simulink model "VSC_GFo_Fixed_Frequency_wi_LCL_v2017b"  (R2017b)
settings: Solver=ode1  StartTime=0.0  StopTime=10  FixedStep=Time_Step  MaxStep=1e-5  RelTol=1e-3
values from neighbouring files (symbols this model uses):
  fb = fn    (= 50)    [VSC_GFo_Init.m]    (also in VSC_GFo_Init_v1.m; VSC_GFo_Init_wi_LCL.m)
  fn = 50    [VSC_GFo_Init.m]    (also in VSC_GFo_Init_v1.m; VSC_GFo_Init_wi_LCL.m)
  GRD00_H = 5    [VSC_GFo_Init.m]    (also in VSC_GFo_Init_v1.m; VSC_GFo_Init_wi_LCL.m)
  GRD00_R = 4/100    (= 0.04)    [VSC_GFo_Init.m]    (also in VSC_GFo_Init_v1.m; VSC_GFo_Init_wi_LCL.m)
  GRD00_TD = 6    [VSC_GFo_Init.m]    (also in VSC_GFo_Init_v1.m = 2; VSC_GFo_Init_wi_LCL.m = 2)
  GRD00_TN = 1    [VSC_GFo_Init.m]    (also in VSC_GFo_Init_v1.m; VSC_GFo_Init_wi_LCL.m)
  GRD00_Ub = GRD00_Un    (= 400000)    [VSC_GFo_Init.m]    (also in VSC_GFo_Init_v1.m; VSC_GFo_Init_wi_LCL.m)
  Time_Step = 40e-6    (= 4e-05)    [VSC_GFo_Init.m]    (also in VSC_GFo_Init_v1.m; VSC_GFo_Init_wi_LCL.m)
  VSC01_Cf_pu = 0.066    [VSC_GFo_Init.m]    (also in VSC_GFo_Init_wi_LCL.m)
  VSC01_Lf_pu = 0.15    [VSC_GFo_Init.m]    (also in VSC_GFo_Init_wi_LCL.m)
  VSC01_Lt_pu = 0.15    [VSC_GFo_Init.m]    (also in VSC_GFo_Init_v1.m; VSC_GFo_Init_wi_LCL.m)
  VSC01_mp1 = 0.0043    [VSC_GFo_Init.m]    (also in VSC_GFo_Init_v1.m; VSC_GFo_Init_wi_LCL.m)
  VSC01_mp2 = 0.003    [VSC_GFo_Init.m]    (also in VSC_GFo_Init_v1.m = 0.0033; VSC_GFo_Init_wi_LCL.m = 0.0033)
  VSC01_mp3 = 0.04    [VSC_GFo_Init.m]    (also in VSC_GFo_Init_v1.m; VSC_GFo_Init_wi_LCL.m)
  VSC01_Pn = 1000 * 1e6    (= 1000000000)    [VSC_GFo_Init.m]    (also in VSC_GFo_Init_v1.m; VSC_GFo_Init_wi_LCL.m)
  VSC01_R = 4/100    (= 0.04)    [VSC_GFo_Init.m]    (also in VSC_GFo_Init_v1.m; VSC_GFo_Init_wi_LCL.m)
  VSC01_Rt_pu = 0.005    [VSC_GFo_Init.m]    (also in VSC_GFo_Init_v1.m; VSC_GFo_Init_wi_LCL.m)
  VSC01_Rv = 0.09    [VSC_GFo_Init.m]    (also in VSC_GFo_Init_v1.m; VSC_GFo_Init_wi_LCL.m)
  VSC01_Sn = VSC01_Pn/VSC01_cosPhi_n    [VSC_GFo_Init.m]    (also in VSC_GFo_Init_v1.m; VSC_GFo_Init_wi_LCL.m)
  VSC01_T1 = 0.121    [VSC_GFo_Init.m]    (also in VSC_GFo_Init_v1.m; VSC_GFo_Init_wi_LCL.m)
  VSC01_T2 = 0.022    [VSC_GFo_Init.m]    (also in VSC_GFo_Init_v1.m; VSC_GFo_Init_wi_LCL.m)
  VSC01_Tr_PLL = 0.010    (= 0.01)    [VSC_GFo_Init.m]    (also in VSC_GFo_Init_v1.m; VSC_GFo_Init_wi_LCL.m)
  VSC01_Udc_n = 640 * 1e3    (= 640000)    [VSC_GFo_Init.m]    (also in VSC_GFo_Init_v1.m; VSC_GFo_Init_wi_LCL.m)
  VSC01_Udcb = VSC01_Udc_n    (= 640000)    [VSC_GFo_Init.m]    (also in VSC_GFo_Init_v1.m; VSC_GFo_Init_wi_LCL.m)
  VSC01_Un1 = 320 * 1e3    (= 320000)    [VSC_GFo_Init.m]    (also in VSC_GFo_Init_v1.m; VSC_GFo_Init_wi_LCL.m)
  VSC01_Un2 = 400 * 1e3    (= 400000)    [VSC_GFo_Init.m]    (also in VSC_GFo_Init_v1.m; VSC_GFo_Init_wi_LCL.m)
  VSC01_W_LF = 60    [VSC_GFo_Init.m]    (also in VSC_GFo_Init_v1.m; VSC_GFo_Init_wi_LCL.m)
  VSC01_wc1 = wb/10    (= 31.4159265359)    [VSC_GFo_Init.m]    (also in VSC_GFo_Init_v1.m; VSC_GFo_Init_wi_LCL.m)
  VSC01_wc2 = 33.3    [VSC_GFo_Init.m]    (also in VSC_GFo_Init_v1.m; VSC_GFo_Init_wi_LCL.m)
  VSC01_wc3 = 2.5    [VSC_GFo_Init.m]    (also in VSC_GFo_Init_v1.m; VSC_GFo_Init_wi_LCL.m)
undefined symbols (not defined in the file or in its folder): C_line, VSC01_id0
libraries: powerlib x31, powerlib_meascontrol x1
(part 3 of 3)

== system VSC_GFo_Fixed_Frequency_wi_LCL_v2017b/VSC00/Strategy 1/Inner controller: Current & Voltage /Current Control/PI current control axis d1 ==
  e : Inport
  x0 : Inport  Port=2
  Damping (d) : Gain  Gain=Kp_i
  Damping (d)1 : Gain  Gain=1/Kp_i
  Integration Time : Gain  Gain=1/Ti_i
  Integrator : Integrator  InitialConditionSource=external
  Sum1 : Sum  Inputs=|++
  Sum2 : Sum  Inputs=-+|
  v_q : Outport
  wires:
  Damping (d)/1 -> v_q/1  "v_d\""
  e/1 -> Integration Time/1, Sum1/2, Sum2/1
  Sum1/1 -> Damping (d)/1
  Integrator/1 -> Sum1/1
  Integration Time/1 -> Integrator/1
  x0/1 -> Damping (d)1/1
  Damping (d)1/1 -> Sum2/2
  Sum2/1 -> Integrator/2

== system VSC_GFo_Fixed_Frequency_wi_LCL_v2017b/VSC00/Strategy 1/Inner controller: Current & Voltage /Voltage Control/PI voltage control axis d ==
  e : Inport
  x0 : Inport  Port=2
  Damping (d) : Gain  Gain=Kp_v
  Damping (d)1 : Gain  Gain=1/Kp_v
  Integration Time : Gain  Gain=1/Ti_iv
  Integrator : Integrator  InitialConditionSource=external
  Sum1 : Sum  Inputs=|++
  Sum2 : Sum  Inputs=-+|
  is_d'' : Outport
  wires:
  Integration Time/1 -> Integrator/1
  Integrator/1 -> Sum1/1
  Sum1/1 -> Damping (d)/1
  Damping (d)/1 -> is_d''/1  "Is_d\""
  Damping (d)1/1 -> Sum2/2
  e/1 -> Sum2/1, Sum1/2, Integration Time/1
  Sum2/1 -> Integrator/2
  x0/1 -> Damping (d)1/1

== system VSC_GFo_Fixed_Frequency_wi_LCL_v2017b/VSC00/Strategy 1/Inner controller: Current & Voltage /Voltage Control/PI voltage control axis d1 ==
  e : Inport
  x0 : Inport  Port=2
  Damping (d) : Gain  Gain=Kp_v
  Damping (d)1 : Gain  Gain=1/Kp_v
  Integration Time : Gain  Gain=1/Ti_iv
  Integrator : Integrator  InitialConditionSource=external
  Sum1 : Sum  Inputs=|++
  Sum2 : Sum  Inputs=-+|
  is_d'' : Outport
  wires:
  Integration Time/1 -> Integrator/1
  Integrator/1 -> Sum1/1
  Sum1/1 -> Damping (d)/1
  Damping (d)/1 -> is_d''/1  "Is_d\""
  Damping (d)1/1 -> Sum2/2
  e/1 -> Sum2/1, Sum1/2, Integration Time/1
  Sum2/1 -> Integrator/2
  x0/1 -> Damping (d)1/1

== system VSC_GFo_Fixed_Frequency_wi_LCL_v2017b/VSC00/Strategy 1/Park Transformation_abc--> dq0/abc --> dq1/abc_alpha_beta_tri4 ==
  a : Inport
  b : Inport  Port=2
  c : Inport  Port=3
  Fcn1 : Fcn  Expr=sqrt(2/3)*(u(1)+u(2)+u(3))
  Fcn3 : Fcn  Expr=sqrt(2/3)*(u(1)-u(2)/2-u(3)/2)
  Fcn5 : Fcn  Expr=(u(2)-u(3))/sqrt(2)
  Mux : Mux  Inputs=3
  Scope5 : Scope
  alpha : Outport
  beta : Outport  Port=2
  wires:
  Fcn5/1 -> beta/1
  Fcn3/1 -> alpha/1
  b/1 -> Mux/2
  a/1 -> Mux/1
  Mux/1 -> Fcn3/1, Fcn1/1, Fcn5/1
  Fcn1/1 -> Scope5/1
  c/1 -> Mux/3

== system VSC_GFo_Fixed_Frequency_wi_LCL_v2017b/VSC00/Strategy 1/Park Transformation_abc--> dq0/abc --> dq1/abc_dq2 ==
  Theta : Inport
  a : Inport  Port=2
  b : Inport  Port=3
  1/Vb1 : Gain  Gain=1/(sqrt(3))
  1/Vb2 : Gain  Gain=1/(sqrt(3))
  Fcn1 : Fcn  Expr=u(2)*cos(u(1))+u(3)*sin(u(1))
  Fcn3 : Fcn  Expr=u(2)*sin(u(1))-u(3)*cos(u(1))
  Mux : Mux  Inputs=3
  d : Outport
  q : Outport  Port=2
  wires:
  1/Vb2/1 -> q/1
  1/Vb1/1 -> d/1
  Fcn1/1 -> 1/Vb2/1
  Fcn3/1 -> 1/Vb1/1
  b/1 -> Mux/3
  a/1 -> Mux/2
  Mux/1 -> Fcn1/1, Fcn3/1
  Theta/1 -> Mux/1

== system VSC_GFo_Fixed_Frequency_wi_LCL_v2017b/VSC00/Strategy 1/Park Transformation_abc--> dq0/abc --> dq2/abc_alpha_beta_tri4 ==
  a : Inport
  b : Inport  Port=2
  c : Inport  Port=3
  Fcn1 : Fcn  Expr=sqrt(2/3)*(u(1)+u(2)+u(3))
  Fcn3 : Fcn  Expr=sqrt(2/3)*(u(1)-u(2)/2-u(3)/2)
  Fcn5 : Fcn  Expr=(u(2)-u(3))/sqrt(2)
  Mux : Mux  Inputs=3
  Scope5 : Scope
  alpha : Outport
  beta : Outport  Port=2
  wires:
  c/1 -> Mux/3
  Fcn1/1 -> Scope5/1
  Mux/1 -> Fcn5/1, Fcn1/1, Fcn3/1
  a/1 -> Mux/1
  b/1 -> Mux/2
  Fcn3/1 -> alpha/1
  Fcn5/1 -> beta/1

== system VSC_GFo_Fixed_Frequency_wi_LCL_v2017b/VSC00/Strategy 1/Park Transformation_abc--> dq0/abc --> dq2/abc_dq2 ==
  Theta : Inport
  a : Inport  Port=2
  b : Inport  Port=3
  1/Vb1 : Gain  Gain=1/(sqrt(3))
  1/Vb2 : Gain  Gain=1/(sqrt(3))
  Fcn1 : Fcn  Expr=u(2)*cos(u(1))+u(3)*sin(u(1))
  Fcn3 : Fcn  Expr=u(2)*sin(u(1))-u(3)*cos(u(1))
  Mux : Mux  Inputs=3
  d : Outport
  q : Outport  Port=2
  wires:
  Theta/1 -> Mux/1
  Mux/1 -> Fcn3/1, Fcn1/1
  a/1 -> Mux/2
  b/1 -> Mux/3
  Fcn3/1 -> 1/Vb1/1
  Fcn1/1 -> 1/Vb2/1
  1/Vb1/1 -> d/1
  1/Vb2/1 -> q/1

== system VSC_GFo_Fixed_Frequency_wi_LCL_v2017b/VSC00/Strategy 1/Park Transformation_abc--> dq0/abc --> dq4/abc_alpha_beta_tri4 ==
  a : Inport
  b : Inport  Port=2
  c : Inport  Port=3
  Fcn1 : Fcn  Expr=sqrt(2/3)*(u(1)+u(2)+u(3))
  Fcn3 : Fcn  Expr=sqrt(2/3)*(u(1)-u(2)/2-u(3)/2)
  Fcn5 : Fcn  Expr=(u(2)-u(3))/sqrt(2)
  Mux : Mux  Inputs=3
  Scope5 : Scope
  alpha : Outport
  beta : Outport  Port=2
  wires:
  c/1 -> Mux/3
  Fcn1/1 -> Scope5/1
  Mux/1 -> Fcn5/1, Fcn1/1, Fcn3/1
  a/1 -> Mux/1
  b/1 -> Mux/2
  Fcn3/1 -> alpha/1
  Fcn5/1 -> beta/1

== system VSC_GFo_Fixed_Frequency_wi_LCL_v2017b/VSC00/Strategy 1/Park Transformation_abc--> dq0/abc --> dq4/abc_dq2 ==
  Theta : Inport
  a : Inport  Port=2
  b : Inport  Port=3
  1/Vb1 : Gain  Gain=1/(sqrt(3))
  1/Vb2 : Gain  Gain=1/(sqrt(3))
  Fcn1 : Fcn  Expr=u(2)*cos(u(1))+u(3)*sin(u(1))
  Fcn3 : Fcn  Expr=u(2)*sin(u(1))-u(3)*cos(u(1))
  Mux : Mux  Inputs=3
  d : Outport
  q : Outport  Port=2
  wires:
  Theta/1 -> Mux/1
  Mux/1 -> Fcn3/1, Fcn1/1
  a/1 -> Mux/2
  b/1 -> Mux/3
  Fcn3/1 -> 1/Vb1/1
  Fcn1/1 -> 1/Vb2/1
  1/Vb1/1 -> d/1
  1/Vb2/1 -> q/1

== system VSC_GFo_Fixed_Frequency_wi_LCL_v2017b/VSC00/Strategy 2/Inner controller: Current & Voltage /Current Control/PI current control axis d ==
  e : Inport
  x0 : Inport  Port=2
  Damping (d) : Gain  Gain=Kp_i
  Damping (d)1 : Gain  Gain=1/Kp_i
  Integration Time : Gain  Gain=1/Ti_i
  Integrator : Integrator  InitialConditionSource=external
  Sum1 : Sum  Inputs=|++
  Sum2 : Sum  Inputs=-+|
  v_d'' : Outport
  wires:
  Damping (d)/1 -> v_d''/1  "v_d"
  e/1 -> Integration Time/1, Sum1/2, Sum2/1
  Sum1/1 -> Damping (d)/1
  Integrator/1 -> Sum1/1
  Integration Time/1 -> Integrator/1
  x0/1 -> Damping (d)1/1
  Damping (d)1/1 -> Sum2/2
  Sum2/1 -> Integrator/2

== system VSC_GFo_Fixed_Frequency_wi_LCL_v2017b/VSC00/Strategy 2/Inner controller: Current & Voltage /Current Control/PI current control axis d1 ==
  e : Inport
  x0 : Inport  Port=2
  Damping (d) : Gain  Gain=Kp_i
  Damping (d)1 : Gain  Gain=1/Kp_i
  Integration Time : Gain  Gain=1/Ti_i
  Integrator : Integrator  InitialConditionSource=external
  Sum1 : Sum  Inputs=|++
  Sum2 : Sum  Inputs=-+|
  v_q : Outport
  wires:
  Damping (d)/1 -> v_q/1  "v_d\""
  e/1 -> Integration Time/1, Sum1/2, Sum2/1
  Sum1/1 -> Damping (d)/1
  Integrator/1 -> Sum1/1
  Integration Time/1 -> Integrator/1
  x0/1 -> Damping (d)1/1
  Damping (d)1/1 -> Sum2/2
  Sum2/1 -> Integrator/2

== system VSC_GFo_Fixed_Frequency_wi_LCL_v2017b/VSC00/Strategy 2/Inner controller: Current & Voltage /Voltage Control/PI voltage control axis d ==
  e : Inport
  x0 : Inport  Port=2
  Damping (d) : Gain  Gain=Kp_v
  Damping (d)1 : Gain  Gain=1/Kp_v
  Integration Time : Gain  Gain=1/Ti_iv
  Integrator : Integrator  InitialConditionSource=external
  Sum1 : Sum  Inputs=|++
  Sum2 : Sum  Inputs=-+|
  is_d'' : Outport
  wires:
  Integration Time/1 -> Integrator/1
  Integrator/1 -> Sum1/1
  Sum1/1 -> Damping (d)/1
  Damping (d)/1 -> is_d''/1  "Is_d\""
  Damping (d)1/1 -> Sum2/2
  e/1 -> Sum2/1, Sum1/2, Integration Time/1
  Sum2/1 -> Integrator/2
  x0/1 -> Damping (d)1/1

== system VSC_GFo_Fixed_Frequency_wi_LCL_v2017b/VSC00/Strategy 2/Inner controller: Current & Voltage /Voltage Control/PI voltage control axis d1 ==
  e : Inport
  x0 : Inport  Port=2
  Damping (d) : Gain  Gain=Kp_v
  Damping (d)1 : Gain  Gain=1/Kp_v
  Integration Time : Gain  Gain=1/Ti_iv
  Integrator : Integrator  InitialConditionSource=external
  Sum1 : Sum  Inputs=|++
  Sum2 : Sum  Inputs=-+|
  is_d'' : Outport
  wires:
  Integration Time/1 -> Integrator/1
  Integrator/1 -> Sum1/1
  Sum1/1 -> Damping (d)/1
  Damping (d)/1 -> is_d''/1  "Is_d\""
  Damping (d)1/1 -> Sum2/2
  e/1 -> Sum2/1, Sum1/2, Integration Time/1
  Sum2/1 -> Integrator/2
  x0/1 -> Damping (d)1/1

== system VSC_GFo_Fixed_Frequency_wi_LCL_v2017b/VSC00/Strategy 2/Park Transformation_abc--> dq0/abc --> dq1/abc_alpha_beta_tri4 ==
  a : Inport
  b : Inport  Port=2
  c : Inport  Port=3
  Fcn1 : Fcn  Expr=sqrt(2/3)*(u(1)+u(2)+u(3))
  Fcn3 : Fcn  Expr=sqrt(2/3)*(u(1)-u(2)/2-u(3)/2)
  Fcn5 : Fcn  Expr=(u(2)-u(3))/sqrt(2)
  Mux : Mux  Inputs=3
  Scope5 : Scope
  alpha : Outport
  beta : Outport  Port=2
  wires:
  Fcn5/1 -> beta/1
  Fcn3/1 -> alpha/1
  b/1 -> Mux/2
  a/1 -> Mux/1
  Mux/1 -> Fcn3/1, Fcn1/1, Fcn5/1
  Fcn1/1 -> Scope5/1
  c/1 -> Mux/3

== system VSC_GFo_Fixed_Frequency_wi_LCL_v2017b/VSC00/Strategy 2/Park Transformation_abc--> dq0/abc --> dq1/abc_dq2 ==
  Theta : Inport
  a : Inport  Port=2
  b : Inport  Port=3
  1/Vb1 : Gain  Gain=1/(sqrt(3))
  1/Vb2 : Gain  Gain=1/(sqrt(3))
  Fcn1 : Fcn  Expr=u(2)*cos(u(1))+u(3)*sin(u(1))
  Fcn3 : Fcn  Expr=u(2)*sin(u(1))-u(3)*cos(u(1))
  Mux : Mux  Inputs=3
  d : Outport
  q : Outport  Port=2
  wires:
  1/Vb2/1 -> q/1
  1/Vb1/1 -> d/1
  Fcn1/1 -> 1/Vb2/1
  Fcn3/1 -> 1/Vb1/1
  b/1 -> Mux/3
  a/1 -> Mux/2
  Mux/1 -> Fcn1/1, Fcn3/1
  Theta/1 -> Mux/1

== system VSC_GFo_Fixed_Frequency_wi_LCL_v2017b/VSC00/Strategy 2/Park Transformation_abc--> dq0/abc --> dq2/abc_alpha_beta_tri4 ==
  a : Inport
  b : Inport  Port=2
  c : Inport  Port=3
  Fcn1 : Fcn  Expr=sqrt(2/3)*(u(1)+u(2)+u(3))
  Fcn3 : Fcn  Expr=sqrt(2/3)*(u(1)-u(2)/2-u(3)/2)
  Fcn5 : Fcn  Expr=(u(2)-u(3))/sqrt(2)
  Mux : Mux  Inputs=3
  Scope5 : Scope
  alpha : Outport
  beta : Outport  Port=2
  wires:
  c/1 -> Mux/3
  Fcn1/1 -> Scope5/1
  Mux/1 -> Fcn5/1, Fcn1/1, Fcn3/1
  a/1 -> Mux/1
  b/1 -> Mux/2
  Fcn3/1 -> alpha/1
  Fcn5/1 -> beta/1

== system VSC_GFo_Fixed_Frequency_wi_LCL_v2017b/VSC00/Strategy 2/Park Transformation_abc--> dq0/abc --> dq2/abc_dq2 ==
  Theta : Inport
  a : Inport  Port=2
  b : Inport  Port=3
  1/Vb1 : Gain  Gain=1/(sqrt(3))
  1/Vb2 : Gain  Gain=1/(sqrt(3))
  Fcn1 : Fcn  Expr=u(2)*cos(u(1))+u(3)*sin(u(1))
  Fcn3 : Fcn  Expr=u(2)*sin(u(1))-u(3)*cos(u(1))
  Mux : Mux  Inputs=3
  d : Outport
  q : Outport  Port=2
  wires:
  Theta/1 -> Mux/1
  Mux/1 -> Fcn3/1, Fcn1/1
  a/1 -> Mux/2
  b/1 -> Mux/3
  Fcn3/1 -> 1/Vb1/1
  Fcn1/1 -> 1/Vb2/1
  1/Vb1/1 -> d/1
  1/Vb2/1 -> q/1

== system VSC_GFo_Fixed_Frequency_wi_LCL_v2017b/VSC00/Strategy 2/Park Transformation_abc--> dq0/abc --> dq4/abc_alpha_beta_tri4 ==
  a : Inport
  b : Inport  Port=2
  c : Inport  Port=3
  Fcn1 : Fcn  Expr=sqrt(2/3)*(u(1)+u(2)+u(3))
  Fcn3 : Fcn  Expr=sqrt(2/3)*(u(1)-u(2)/2-u(3)/2)
  Fcn5 : Fcn  Expr=(u(2)-u(3))/sqrt(2)
  Mux : Mux  Inputs=3
  Scope5 : Scope
  alpha : Outport
  beta : Outport  Port=2
  wires:
  c/1 -> Mux/3
  Fcn1/1 -> Scope5/1
  Mux/1 -> Fcn5/1, Fcn1/1, Fcn3/1
  a/1 -> Mux/1
  b/1 -> Mux/2
  Fcn3/1 -> alpha/1
  Fcn5/1 -> beta/1

== system VSC_GFo_Fixed_Frequency_wi_LCL_v2017b/VSC00/Strategy 2/Park Transformation_abc--> dq0/abc --> dq4/abc_dq2 ==
  Theta : Inport
  a : Inport  Port=2
  b : Inport  Port=3
  1/Vb1 : Gain  Gain=1/(sqrt(3))
  1/Vb2 : Gain  Gain=1/(sqrt(3))
  Fcn1 : Fcn  Expr=u(2)*cos(u(1))+u(3)*sin(u(1))
  Fcn3 : Fcn  Expr=u(2)*sin(u(1))-u(3)*cos(u(1))
  Mux : Mux  Inputs=3
  d : Outport
  q : Outport  Port=2
  wires:
  Theta/1 -> Mux/1
  Mux/1 -> Fcn3/1, Fcn1/1
  a/1 -> Mux/2
  b/1 -> Mux/3
  Fcn3/1 -> 1/Vb1/1
  Fcn1/1 -> 1/Vb2/1
  1/Vb1/1 -> d/1
  1/Vb2/1 -> q/1

== system VSC_GFo_Fixed_Frequency_wi_LCL_v2017b/VSC00/Strategy 3/Inner controller: Current & Voltage /Current Control/PI current control axis d ==
  e : Inport
  x0 : Inport  Port=2
  Damping (d) : Gain  Gain=Kp_i
  Damping (d)1 : Gain  Gain=1/Kp_i
  Integration Time : Gain  Gain=1/Ti_i
  Integrator : Integrator  InitialConditionSource=external
  Sum1 : Sum  Inputs=|++
  Sum2 : Sum  Inputs=-+|
  v_d'' : Outport
  wires:
  Damping (d)/1 -> v_d''/1  "v_d"
  e/1 -> Integration Time/1, Sum1/2, Sum2/1
  Sum1/1 -> Damping (d)/1
  Integrator/1 -> Sum1/1
  Integration Time/1 -> Integrator/1
  x0/1 -> Damping (d)1/1
  Damping (d)1/1 -> Sum2/2
  Sum2/1 -> Integrator/2

== system VSC_GFo_Fixed_Frequency_wi_LCL_v2017b/VSC00/Strategy 3/Inner controller: Current & Voltage /Current Control/PI current control axis d1 ==
  e : Inport
  x0 : Inport  Port=2
  Damping (d) : Gain  Gain=Kp_i
  Damping (d)1 : Gain  Gain=1/Kp_i
  Integration Time : Gain  Gain=1/Ti_i
  Integrator : Integrator  InitialConditionSource=external
  Sum1 : Sum  Inputs=|++
  Sum2 : Sum  Inputs=-+|
  v_q : Outport
  wires:
  Damping (d)/1 -> v_q/1  "v_d\""
  e/1 -> Integration Time/1, Sum1/2, Sum2/1
  Sum1/1 -> Damping (d)/1
  Integrator/1 -> Sum1/1
  Integration Time/1 -> Integrator/1
  x0/1 -> Damping (d)1/1
  Damping (d)1/1 -> Sum2/2
  Sum2/1 -> Integrator/2

== system VSC_GFo_Fixed_Frequency_wi_LCL_v2017b/VSC00/Strategy 3/Inner controller: Current & Voltage /Voltage Control/PI voltage control axis d ==
  e : Inport
  x0 : Inport  Port=2
  Damping (d) : Gain  Gain=Kp_v
  Damping (d)1 : Gain  Gain=1/Kp_v
  Integration Time : Gain  Gain=1/Ti_iv
  Integrator : Integrator  InitialConditionSource=external
  Sum1 : Sum  Inputs=|++
  Sum2 : Sum  Inputs=-+|
  is_d'' : Outport
  wires:
  Integration Time/1 -> Integrator/1
  Integrator/1 -> Sum1/1
  Sum1/1 -> Damping (d)/1
  Damping (d)/1 -> is_d''/1  "Is_d\""
  Damping (d)1/1 -> Sum2/2
  e/1 -> Sum2/1, Sum1/2, Integration Time/1
  Sum2/1 -> Integrator/2
  x0/1 -> Damping (d)1/1

== system VSC_GFo_Fixed_Frequency_wi_LCL_v2017b/VSC00/Strategy 3/Inner controller: Current & Voltage /Voltage Control/PI voltage control axis d1 ==
  e : Inport
  x0 : Inport  Port=2
  Damping (d) : Gain  Gain=Kp_v
  Damping (d)1 : Gain  Gain=1/Kp_v
  Integration Time : Gain  Gain=1/Ti_iv
  Integrator : Integrator  InitialConditionSource=external
  Sum1 : Sum  Inputs=|++
  Sum2 : Sum  Inputs=-+|
  is_d'' : Outport
  wires:
  Integration Time/1 -> Integrator/1
  Integrator/1 -> Sum1/1
  Sum1/1 -> Damping (d)/1
  Damping (d)/1 -> is_d''/1  "Is_d\""
  Damping (d)1/1 -> Sum2/2
  e/1 -> Sum2/1, Sum1/2, Integration Time/1
  Sum2/1 -> Integrator/2
  x0/1 -> Damping (d)1/1

== system VSC_GFo_Fixed_Frequency_wi_LCL_v2017b/VSC00/Strategy 3/Park Transformation_abc--> dq0/abc --> dq1/abc_alpha_beta_tri4 ==
  a : Inport
  b : Inport  Port=2
  c : Inport  Port=3
  Fcn1 : Fcn  Expr=sqrt(2/3)*(u(1)+u(2)+u(3))
  Fcn3 : Fcn  Expr=sqrt(2/3)*(u(1)-u(2)/2-u(3)/2)
  Fcn5 : Fcn  Expr=(u(2)-u(3))/sqrt(2)
  Mux : Mux  Inputs=3
  Scope5 : Scope
  alpha : Outport
  beta : Outport  Port=2
  wires:
  Fcn5/1 -> beta/1
  Fcn3/1 -> alpha/1
  b/1 -> Mux/2
  a/1 -> Mux/1
  Mux/1 -> Fcn3/1, Fcn1/1, Fcn5/1
  Fcn1/1 -> Scope5/1
  c/1 -> Mux/3

== system VSC_GFo_Fixed_Frequency_wi_LCL_v2017b/VSC00/Strategy 3/Park Transformation_abc--> dq0/abc --> dq1/abc_dq2 ==
  Theta : Inport
  a : Inport  Port=2
  b : Inport  Port=3
  1/Vb1 : Gain  Gain=1/(sqrt(3))
  1/Vb2 : Gain  Gain=1/(sqrt(3))
  Fcn1 : Fcn  Expr=u(2)*cos(u(1))+u(3)*sin(u(1))
  Fcn3 : Fcn  Expr=u(2)*sin(u(1))-u(3)*cos(u(1))
  Mux : Mux  Inputs=3
  d : Outport
  q : Outport  Port=2
  wires:
  1/Vb2/1 -> q/1
  1/Vb1/1 -> d/1
  Fcn1/1 -> 1/Vb2/1
  Fcn3/1 -> 1/Vb1/1
  b/1 -> Mux/3
  a/1 -> Mux/2
  Mux/1 -> Fcn1/1, Fcn3/1
  Theta/1 -> Mux/1

== system VSC_GFo_Fixed_Frequency_wi_LCL_v2017b/VSC00/Strategy 3/Park Transformation_abc--> dq0/abc --> dq2/abc_alpha_beta_tri4 ==
  a : Inport
  b : Inport  Port=2
  c : Inport  Port=3
  Fcn1 : Fcn  Expr=sqrt(2/3)*(u(1)+u(2)+u(3))
  Fcn3 : Fcn  Expr=sqrt(2/3)*(u(1)-u(2)/2-u(3)/2)
  Fcn5 : Fcn  Expr=(u(2)-u(3))/sqrt(2)
  Mux : Mux  Inputs=3
  Scope5 : Scope
  alpha : Outport
  beta : Outport  Port=2
  wires:
  c/1 -> Mux/3
  Fcn1/1 -> Scope5/1
  Mux/1 -> Fcn5/1, Fcn1/1, Fcn3/1
  a/1 -> Mux/1
  b/1 -> Mux/2
  Fcn3/1 -> alpha/1
  Fcn5/1 -> beta/1

== system VSC_GFo_Fixed_Frequency_wi_LCL_v2017b/VSC00/Strategy 3/Park Transformation_abc--> dq0/abc --> dq2/abc_dq2 ==
  Theta : Inport
  a : Inport  Port=2
  b : Inport  Port=3
  1/Vb1 : Gain  Gain=1/(sqrt(3))
  1/Vb2 : Gain  Gain=1/(sqrt(3))
  Fcn1 : Fcn  Expr=u(2)*cos(u(1))+u(3)*sin(u(1))
  Fcn3 : Fcn  Expr=u(2)*sin(u(1))-u(3)*cos(u(1))
  Mux : Mux  Inputs=3
  d : Outport
  q : Outport  Port=2
  wires:
  Theta/1 -> Mux/1
  Mux/1 -> Fcn3/1, Fcn1/1
  a/1 -> Mux/2
  b/1 -> Mux/3
  Fcn3/1 -> 1/Vb1/1
  Fcn1/1 -> 1/Vb2/1
  1/Vb1/1 -> d/1
  1/Vb2/1 -> q/1

== system VSC_GFo_Fixed_Frequency_wi_LCL_v2017b/VSC00/Strategy 3/Park Transformation_abc--> dq0/abc --> dq4/abc_alpha_beta_tri4 ==
  a : Inport
  b : Inport  Port=2
  c : Inport  Port=3
  Fcn1 : Fcn  Expr=sqrt(2/3)*(u(1)+u(2)+u(3))
  Fcn3 : Fcn  Expr=sqrt(2/3)*(u(1)-u(2)/2-u(3)/2)
  Fcn5 : Fcn  Expr=(u(2)-u(3))/sqrt(2)
  Mux : Mux  Inputs=3
  Scope5 : Scope
  alpha : Outport
  beta : Outport  Port=2
  wires:
  c/1 -> Mux/3
  Fcn1/1 -> Scope5/1
  Mux/1 -> Fcn5/1, Fcn1/1, Fcn3/1
  a/1 -> Mux/1
  b/1 -> Mux/2
  Fcn3/1 -> alpha/1
  Fcn5/1 -> beta/1

== system VSC_GFo_Fixed_Frequency_wi_LCL_v2017b/VSC00/Strategy 3/Park Transformation_abc--> dq0/abc --> dq4/abc_dq2 ==
  Theta : Inport
  a : Inport  Port=2
  b : Inport  Port=3
  1/Vb1 : Gain  Gain=1/(sqrt(3))
  1/Vb2 : Gain  Gain=1/(sqrt(3))
  Fcn1 : Fcn  Expr=u(2)*cos(u(1))+u(3)*sin(u(1))
  Fcn3 : Fcn  Expr=u(2)*sin(u(1))-u(3)*cos(u(1))
  Mux : Mux  Inputs=3
  d : Outport
  q : Outport  Port=2
  wires:
  Theta/1 -> Mux/1
  Mux/1 -> Fcn3/1, Fcn1/1
  a/1 -> Mux/2
  b/1 -> Mux/3
  Fcn3/1 -> 1/Vb1/1
  Fcn1/1 -> 1/Vb2/1
  1/Vb1/1 -> d/1
  1/Vb2/1 -> q/1

== system VSC_GFo_Fixed_Frequency_wi_LCL_v2017b/Voltage Source/Voltage generation/Voltage generation/dq  -->  abc /abc_alpha_beta ==
  a : Inport
  b : Inport  Port=2
  Fcn1 : Fcn  Expr=(-u(1)-sqrt(3)*u(2))/2
  Fcn3 : Fcn  Expr=u(1)
  Fcn5 : Fcn  Expr=(-u(1)+sqrt(3)*u(2))/2
  Gain1 : Gain  Gain=sqrt(2)
  Gain2 : Gain  Gain=sqrt(2)
  Gain3 : Gain  Gain=sqrt(2)
  Mux : Mux  Inputs=2
  a1 : Outport
  b1 : Outport  Port=2
  c : Outport  Port=3
  wires:
  Mux/1 -> Fcn5/1, Fcn1/1, Fcn3/1
  a/1 -> Mux/1
  b/1 -> Mux/2
  Fcn3/1 -> Gain3/1
  Fcn5/1 -> Gain2/1
  Fcn1/1 -> Gain1/1
  Gain1/1 -> c/1
  Gain2/1 -> b1/1
  Gain3/1 -> a1/1

== system VSC_GFo_Fixed_Frequency_wi_LCL_v2017b/Voltage Source/Voltage generation/Voltage generation/dq  -->  abc /abc_dq2 ==
  Theta : Inport
  d : Inport  Port=2
  q : Inport  Port=3
  Fcn1 : Fcn  Expr=-u(2)*cos(u(1))+u(3)*sin(u(1))
  Fcn3 : Fcn  Expr=u(2)*sin(u(1))+u(3)*cos(u(1))
  Mux : Mux  Inputs=3
  a : Outport
  b : Outport  Port=2
  wires:
  Fcn1/1 -> b/1
  Fcn3/1 -> a/1
  q/1 -> Mux/3
  d/1 -> Mux/2
  Theta/1 -> Mux/1
  Mux/1 -> Fcn3/1, Fcn1/1
